simulink model "newBLDCmodel_r2018a"  (R2018a)
settings: Solver=ode4  StartTime=0.0  StopTime=200  FixedStep=.01  MaxStep=.001  RelTol=1e-3
libraries: simulink x8
settings Model: Creator=tdarrah  LastModifiedBy=tdarrah
settings SolverCC: InitialStep=.001  ShapePreserveControl=EnableAll
settings CodeAppCC: StateflowObjectComments=on

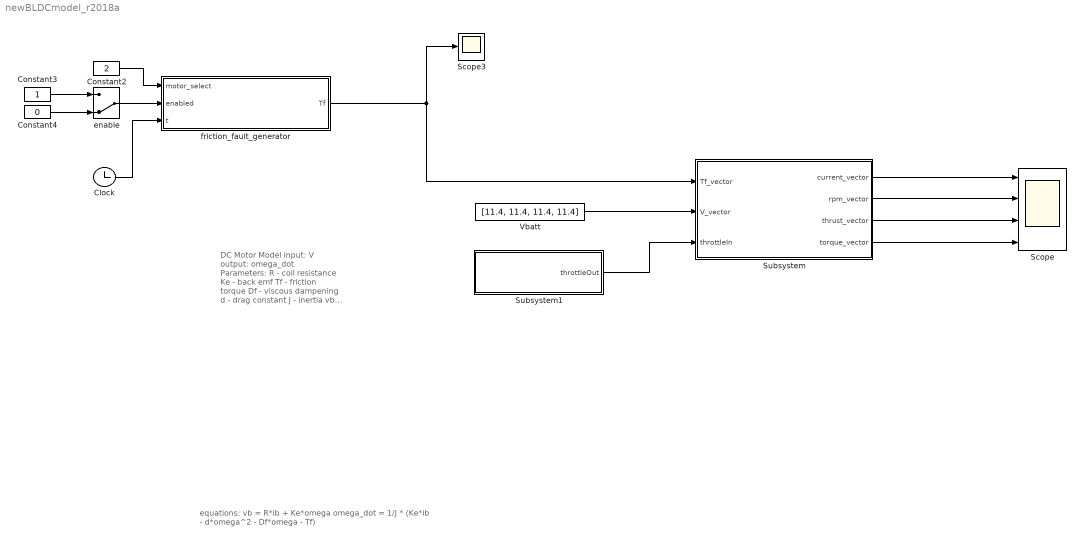
== system newBLDCmodel_r2018a ==
  note: equations:
      |
      | vb = R*ib + Ke*omega
      | omega_dot = 1/J * (Ke*ib - d*omega^2 - Df*omega - Tf)
  note: DC Motor Model
      |
      | input:
      | V
      |
      | output:
      | omega_dot
      |
      | Parameters:
      | R   - coil resistance
      | Ke - back emf
      | Tf  - friction torque
      | Df  - viscous dampening
      | d   - drag constant
      | J   - inertia
      | vb - average battery voltage
      | ib  - average battery current
  Clock : Clock
  Constant2 : Constant  Value=2
  Constant3 : Constant
  Constant4 : Constant  Value=0
  Scope : Scope  NumInputPorts=4
  Scope3 : Scope
  Subsystem : Subsystem
  Subsystem1 : Subsystem
  Vbatt : Constant  Value=[11.4, 11.4, 11.4, 11.4]
  enable : ManualSwitch  CurrentSetting=0
  friction_fault_generator : MATLAB Function  TreatAsAtomicUnit=on
  wires:
  Constant3/1 -> enable/1
  Constant4/1 -> enable/2
  Constant2/1 -> friction_fault_generator/1(motor_select)
  enable/1 -> friction_fault_generator/2(enabled)
  Clock/1 -> friction_fault_generator/3(t)
  friction_fault_generator/1(Tf) -> Subsystem/1(Tf_vector), Scope3/1
  Vbatt/1 -> Subsystem/2(V_vector)
  Subsystem/1(current_vector) -> Scope/1
  Subsystem/2(rpm_vector) -> Scope/2
  Subsystem/3(thrust_vector) -> Scope/3
  Subsystem/4(torque_vector) -> Scope/4
  Subsystem1/1(throttleOut) -> Subsystem/3(throttleIn)

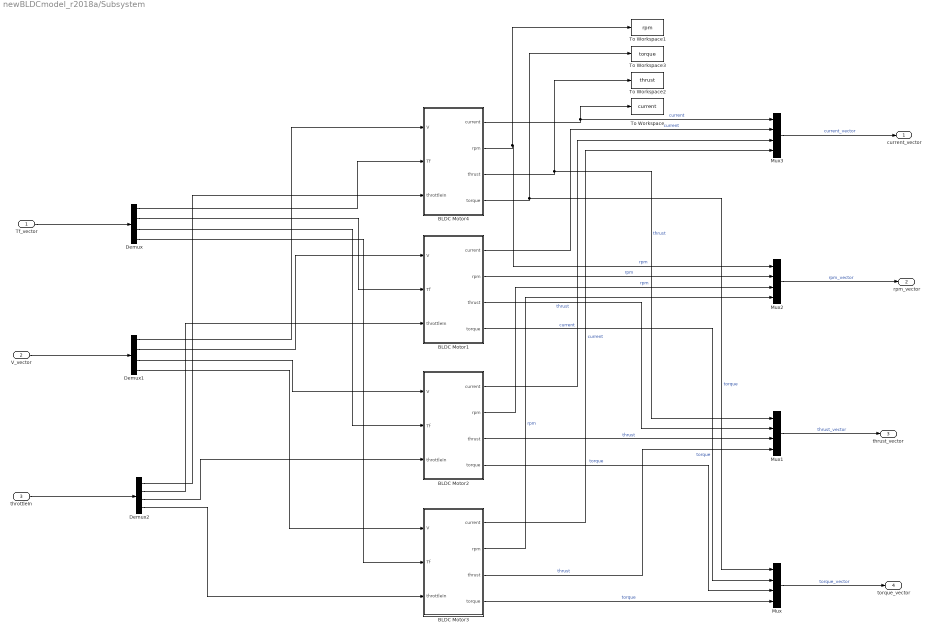
== system newBLDCmodel_r2018a/Subsystem ==
  Tf_vector : Inport
  V_vector : Inport  Port=2
  throttleIn : Inport  Port=3
  BLDC Motor1 : Subsystem
  BLDC Motor2 : Subsystem
  BLDC Motor3 : Subsystem
  BLDC Motor4 : Subsystem
  Demux : Demux
  Demux1 : Demux
  Demux2 : Demux
  Mux{,1..3} (4 alike) : Mux
  To Workspace : ToWorkspace  VariableName=current  SaveFormat=Timeseries  SampleTime=-1
  To Workspace1 : ToWorkspace  VariableName=rpm  SaveFormat=Timeseries  SampleTime=-1
  To Workspace2 : ToWorkspace  VariableName=thrust  SaveFormat=Timeseries  SampleTime=-1
  To Workspace3 : ToWorkspace  VariableName=torque  SaveFormat=Timeseries  SampleTime=-1
  current_vector : Outport
  rpm_vector : Outport  Port=2
  thrust_vector : Outport  Port=3
  torque_vector : Outport  Port=4
  wires:
  BLDC Motor4/2(rpm) -> To Workspace1/1, Mux2/1  "rpm"
  Demux1/3 -> BLDC Motor2/1(V)
  BLDC Motor4/1(current) -> To Workspace/1, Mux3/1  "current"
  BLDC Motor3/3(thrust) -> Mux1/4  "thrust"
  V_vector/1 -> Demux1/1
  Demux1/2 -> BLDC Motor1/1(V)
  BLDC Motor4/3(thrust) -> To Workspace2/1, Mux1/1  "thrust"
  Demux1/4 -> BLDC Motor3/1(V)
  BLDC Motor4/4(torque) -> To Workspace3/1, Mux/1  "torque"
  Mux2/1 -> rpm_vector/1  "rpm_vector"
  Demux/2 -> BLDC Motor1/2(Tf)
  BLDC Motor2/3(thrust) -> Mux1/3  "thrust"
  BLDC Motor1/1(current) -> Mux3/2  "current"
  Tf_vector/1 -> Demux/1
  Demux/1 -> BLDC Motor4/2(Tf)
  BLDC Motor2/1(current) -> Mux3/3  "current"
  Mux3/1 -> current_vector/1  "current_vector"
  BLDC Motor1/3(thrust) -> Mux1/2  "thrust"
  Mux1/1 -> thrust_vector/1  "thrust_vector"
  BLDC Motor2/2(rpm) -> Mux2/3  "rpm"
  Demux/4 -> BLDC Motor3/2(Tf)
  BLDC Motor2/4(torque) -> Mux/3  "torque"
  BLDC Motor1/2(rpm) -> Mux2/2  "rpm"
  Mux/1 -> torque_vector/1  "torque_vector"
  Demux/3 -> BLDC Motor2/2(Tf)
  BLDC Motor1/4(torque) -> Mux/2  "torque"
  BLDC Motor3/1(current) -> Mux3/4  "current"
  Demux1/1 -> BLDC Motor4/1(V)
  BLDC Motor3/4(torque) -> Mux/4  "torque"
  BLDC Motor3/2(rpm) -> Mux2/4  "rpm"
  throttleIn/1 -> Demux2/1
  Demux2/1 -> BLDC Motor4/3(throttleIn)
  Demux2/2 -> BLDC Motor1/3(throttleIn)
  Demux2/3 -> BLDC Motor2/3(throttleIn)
  Demux2/4 -> BLDC Motor3/3(throttleIn)

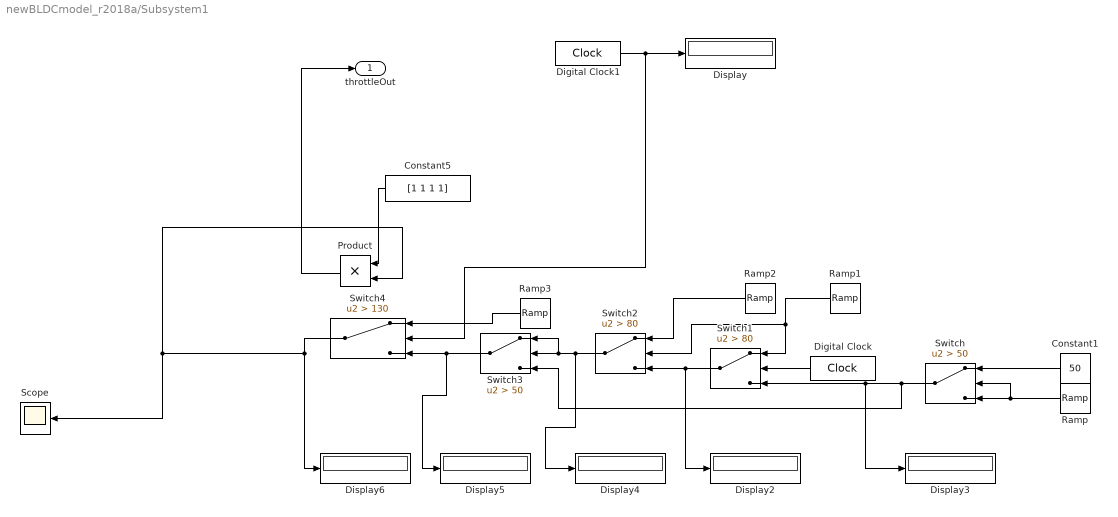
== system newBLDCmodel_r2018a/Subsystem1 ==
  Constant1 : Constant  Value=50
  Constant5 : Constant  Value=[1 1 1 1]
  Digital Clock : DigitalClock
  Digital Clock1 : DigitalClock
  Display{,2..6} (6 alike) : Display
  Product : Product
  Ramp : simulink/Sources/Ramp  slope=1  start=0  InitialOutput=0
  Ramp1 : simulink/Sources/Ramp  slope=2  start=80  InitialOutput=50
  Ramp2 : simulink/Sources/Ramp  slope=-2  start=100  InitialOutput=80
  Ramp3 : simulink/Sources/Ramp  slope=-.63  start=130  InitialOutput=50
  Scope : Scope
  Switch : Switch  Criteria=u2 > Threshold  Threshold=50
  Switch1 : Switch  Criteria=u2 > Threshold  Threshold=80
  Switch2 : Switch  Criteria=u2 > Threshold  Threshold=80
  Switch3 : Switch  Criteria=u2 > Threshold  Threshold=50
  Switch4 : Switch  Criteria=u2 > Threshold  Threshold=130
  throttleOut : Outport
  wires:
  Constant1/1 -> Switch/1
  Product/1 -> throttleOut/1
  Ramp/1 -> Switch/2, Switch/3
  Constant5/1 -> Product/1
  Switch/1 -> Switch3/3, Display3/1, Switch1/3
  Digital Clock/1 -> Switch1/2
  Ramp1/1 -> Switch2/2, Switch1/1
  Switch1/1 -> Display2/1, Switch2/3
  Ramp2/1 -> Switch2/1
  Digital Clock1/1 -> Switch4/2, Display/1
  Switch2/1 -> Display4/1, Switch3/1, Switch3/2
  Switch3/1 -> Display5/1, Switch4/3
  Ramp3/1 -> Switch4/1
  Switch4/1 -> Scope/1, Product/2, Display6/1

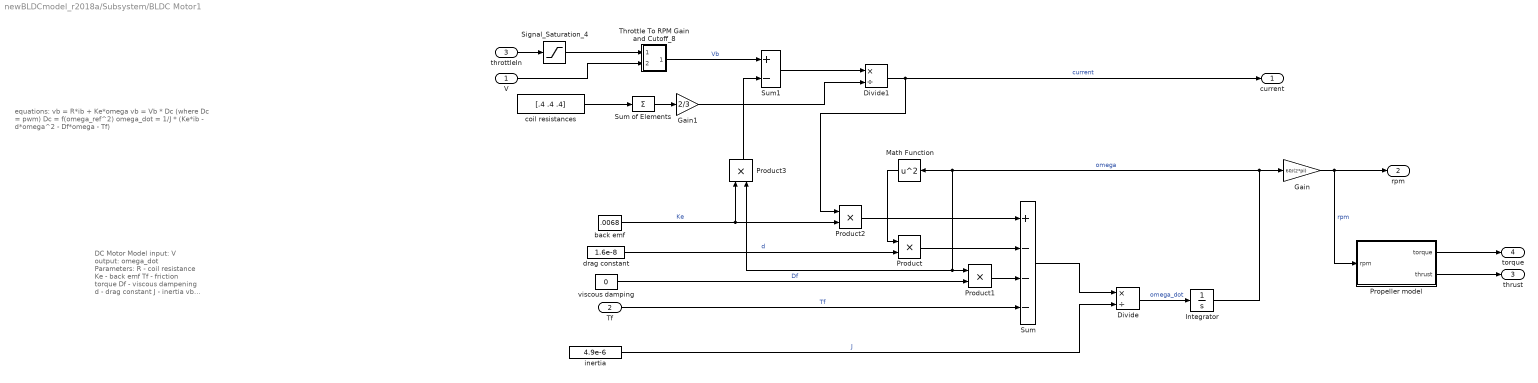
== system newBLDCmodel_r2018a/Subsystem/BLDC Motor1 ==
  note: DC Motor Model
      |
      | input:
      | V
      |
      | output:
      | omega_dot
      |
      | Parameters:
      | R   - coil resistance
      | Ke - back emf
      | Tf  - friction torque
      | Df  - viscous dampening
      | d   - drag constant
      | J   - inertia
      |
      |
      | vb - average battery voltage
      | ib  - average battery current
  note: equations:
      |
      | vb = R*ib + Ke*omega
      | vb = Vb * Dc  (where Dc = pwm)
      | Dc = f(omega_ref^2)
      |
      | omega_dot = 1/J * (Ke*ib - d*omega^2 - Df*omega - Tf)
  V : Inport
  Tf : Inport  Port=2
  throttleIn : Inport  Port=3
  Divide : Product  Inputs=*/
  Divide1 : Product  Inputs=*/
  Gain : Gain  Gain=60/(2*pi)
  Gain1 : Gain  Gain=2/3
  Integrator : Integrator
  Math Function : Math  Operator=square  SaturateOnIntegerOverflow=on
  Product{,1..3} (4 alike) : Product
  "Propeller model " : MATLAB Function  TreatAsAtomicUnit=on
  Signal_Saturation_4 : Saturate  UpperLimit=100  LowerLimit=0
  Sum : Sum  Inputs=+---
  Sum of Elements : Sum  Inputs=+
  Sum1 : Sum  Inputs=+-
  Throttle To RPM Gain and Cutoff_8 : Subsystem
  back emf : Constant  Value=.0068
  coil resistances : Constant  Value=[.4 .4 .4]
  drag constant : Constant  Value=1.6e-8
  inertia : Constant  Value=4.9e-6
  viscous damping : Constant  Value=0
  current : Outport
  rpm : Outport  Port=2
  thrust : Outport  Port=3
  torque : Outport  Port=4
  wires:
  Divide/1 -> Integrator/1  "omega_dot"
  Integrator/1 -> Math Function/1, Product1/1, Product3/2, Gain/1  "omega"
  Gain/1 -> rpm/1, "Propeller model "/1(rpm)  "rpm"
  inertia/1 -> Divide/2  "J"
  drag constant/1 -> Product/2  "d"
  Math Function/1 -> Product/1
  viscous damping/1 -> Product1/2  "Df"
  Tf/1 -> Sum/4  "Tf"
  back emf/1 -> Product3/1, Product2/2  "Ke"
  Product2/1 -> Sum/1
  Divide1/1 -> Product2/1, current/1  "current"
  V/1 -> Throttle To RPM Gain and Cutoff_8/2(Vs)
  Product3/1 -> Sum1/2
  Sum1/1 -> Divide1/1
  Gain1/1 -> Divide1/2
  "Propeller model "/2(thrust) -> thrust/1
  "Propeller model "/1(torque) -> torque/1
  Product1/1 -> Sum/3
  Product/1 -> Sum/2
  Sum/1 -> Divide/1
  coil resistances/1 -> Sum of Elements/1
  Sum of Elements/1 -> Gain1/1
  throttleIn/1 -> Signal_Saturation_4/1
  Signal_Saturation_4/1 -> Throttle To RPM Gain and Cutoff_8/1(In5)
  Throttle To RPM Gain and Cutoff_8/1(Out5) -> Sum1/1  "Vb"

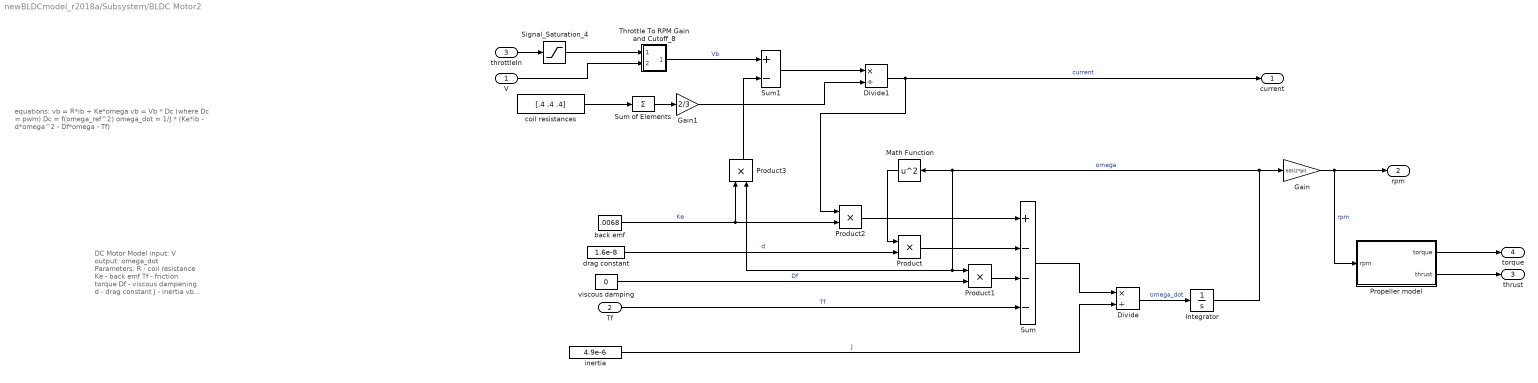
== system newBLDCmodel_r2018a/Subsystem/BLDC Motor2 ==
  note: DC Motor Model
      |
      | input:
      | V
      |
      | output:
      | omega_dot
      |
      | Parameters:
      | R   - coil resistance
      | Ke - back emf
      | Tf  - friction torque
      | Df  - viscous dampening
      | d   - drag constant
      | J   - inertia
      |
      |
      | vb - average battery voltage
      | ib  - average battery current
  note: equations:
      |
      | vb = R*ib + Ke*omega
      | vb = Vb * Dc  (where Dc = pwm)
      | Dc = f(omega_ref^2)
      |
      | omega_dot = 1/J * (Ke*ib - d*omega^2 - Df*omega - Tf)
  V : Inport
  Tf : Inport  Port=2
  throttleIn : Inport  Port=3
  Divide : Product  Inputs=*/
  Divide1 : Product  Inputs=*/
  Gain : Gain  Gain=60/(2*pi)
  Gain1 : Gain  Gain=2/3
  Integrator : Integrator
  Math Function : Math  Operator=square  SaturateOnIntegerOverflow=on
  Product{,1..3} (4 alike) : Product
  "Propeller model " : MATLAB Function  TreatAsAtomicUnit=on
  Signal_Saturation_4 : Saturate  UpperLimit=100  LowerLimit=0
  Sum : Sum  Inputs=+---
  Sum of Elements : Sum  Inputs=+
  Sum1 : Sum  Inputs=+-
  Throttle To RPM Gain and Cutoff_8 : Subsystem
  back emf : Constant  Value=.0068
  coil resistances : Constant  Value=[.4 .4 .4]
  drag constant : Constant  Value=1.6e-8
  inertia : Constant  Value=4.9e-6
  viscous damping : Constant  Value=0
  current : Outport
  rpm : Outport  Port=2
  thrust : Outport  Port=3
  torque : Outport  Port=4
  wires:
  Divide/1 -> Integrator/1  "omega_dot"
  Integrator/1 -> Math Function/1, Product1/1, Product3/2, Gain/1  "omega"
  Gain/1 -> rpm/1, "Propeller model "/1(rpm)  "rpm"
  inertia/1 -> Divide/2  "J"
  drag constant/1 -> Product/2  "d"
  Math Function/1 -> Product/1
  viscous damping/1 -> Product1/2  "Df"
  Tf/1 -> Sum/4  "Tf"
  back emf/1 -> Product3/1, Product2/2  "Ke"
  Product2/1 -> Sum/1
  Divide1/1 -> Product2/1, current/1  "current"
  V/1 -> Throttle To RPM Gain and Cutoff_8/2(Vs)
  Product3/1 -> Sum1/2
  Sum1/1 -> Divide1/1
  Gain1/1 -> Divide1/2
  "Propeller model "/2(thrust) -> thrust/1
  "Propeller model "/1(torque) -> torque/1
  Product1/1 -> Sum/3
  Product/1 -> Sum/2
  Sum/1 -> Divide/1
  coil resistances/1 -> Sum of Elements/1
  Sum of Elements/1 -> Gain1/1
  throttleIn/1 -> Signal_Saturation_4/1
  Signal_Saturation_4/1 -> Throttle To RPM Gain and Cutoff_8/1(In5)
  Throttle To RPM Gain and Cutoff_8/1(Out5) -> Sum1/1  "Vb"

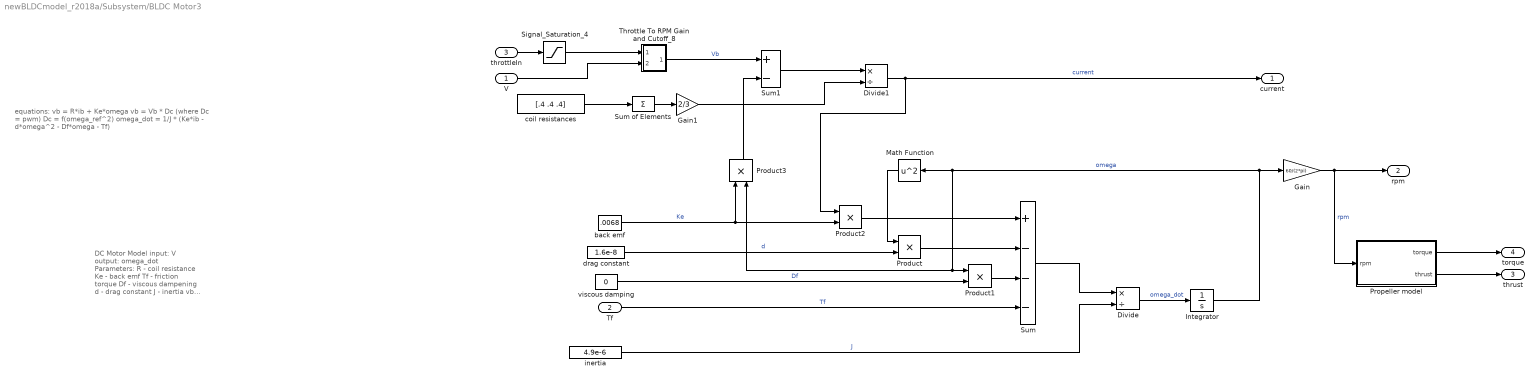
== system newBLDCmodel_r2018a/Subsystem/BLDC Motor3 ==
  note: DC Motor Model
      |
      | input:
      | V
      |
      | output:
      | omega_dot
      |
      | Parameters:
      | R   - coil resistance
      | Ke - back emf
      | Tf  - friction torque
      | Df  - viscous dampening
      | d   - drag constant
      | J   - inertia
      |
      |
      | vb - average battery voltage
      | ib  - average battery current
  note: equations:
      |
      | vb = R*ib + Ke*omega
      | vb = Vb * Dc  (where Dc = pwm)
      | Dc = f(omega_ref^2)
      |
      | omega_dot = 1/J * (Ke*ib - d*omega^2 - Df*omega - Tf)
  V : Inport
  Tf : Inport  Port=2
  throttleIn : Inport  Port=3
  Divide : Product  Inputs=*/
  Divide1 : Product  Inputs=*/
  Gain : Gain  Gain=60/(2*pi)
  Gain1 : Gain  Gain=2/3
  Integrator : Integrator
  Math Function : Math  Operator=square  SaturateOnIntegerOverflow=on
  Product{,1..3} (4 alike) : Product
  "Propeller model " : MATLAB Function  TreatAsAtomicUnit=on
  Signal_Saturation_4 : Saturate  UpperLimit=100  LowerLimit=0
  Sum : Sum  Inputs=+---
  Sum of Elements : Sum  Inputs=+
  Sum1 : Sum  Inputs=+-
  Throttle To RPM Gain and Cutoff_8 : Subsystem
  back emf : Constant  Value=.0068
  coil resistances : Constant  Value=[.4 .4 .4]
  drag constant : Constant  Value=1.6e-8
  inertia : Constant  Value=4.9e-6
  viscous damping : Constant  Value=0
  current : Outport
  rpm : Outport  Port=2
  thrust : Outport  Port=3
  torque : Outport  Port=4
  wires:
  Divide/1 -> Integrator/1  "omega_dot"
  Integrator/1 -> Math Function/1, Product1/1, Product3/2, Gain/1  "omega"
  Gain/1 -> rpm/1, "Propeller model "/1(rpm)  "rpm"
  inertia/1 -> Divide/2  "J"
  drag constant/1 -> Product/2  "d"
  Math Function/1 -> Product/1
  viscous damping/1 -> Product1/2  "Df"
  Tf/1 -> Sum/4  "Tf"
  back emf/1 -> Product3/1, Product2/2  "Ke"
  Product2/1 -> Sum/1
  Divide1/1 -> Product2/1, current/1  "current"
  V/1 -> Throttle To RPM Gain and Cutoff_8/2(Vs)
  Product3/1 -> Sum1/2
  Sum1/1 -> Divide1/1
  Gain1/1 -> Divide1/2
  "Propeller model "/2(thrust) -> thrust/1
  "Propeller model "/1(torque) -> torque/1
  Product1/1 -> Sum/3
  Product/1 -> Sum/2
  Sum/1 -> Divide/1
  coil resistances/1 -> Sum of Elements/1
  Sum of Elements/1 -> Gain1/1
  throttleIn/1 -> Signal_Saturation_4/1
  Signal_Saturation_4/1 -> Throttle To RPM Gain and Cutoff_8/1(In5)
  Throttle To RPM Gain and Cutoff_8/1(Out5) -> Sum1/1  "Vb"

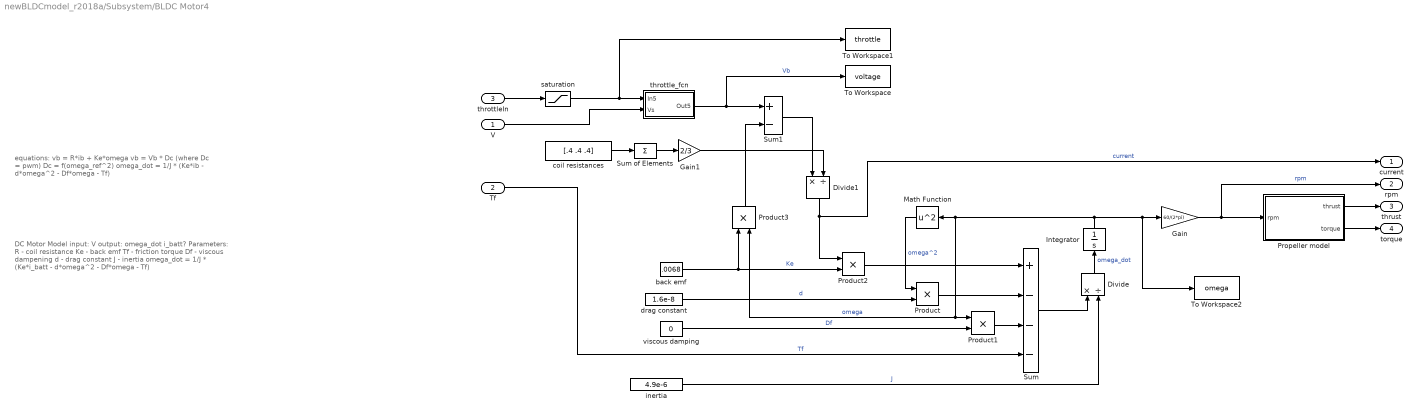
== system newBLDCmodel_r2018a/Subsystem/BLDC Motor4 ==
  note: DC Motor Model
      |
      | input:
      | V
      |
      | output:
      | omega_dot
      | i_batt?
      |
      |
      | Parameters:
      | R   - coil resistance
      | Ke - back emf
      | Tf  - friction torque
      | Df  - viscous dampening
      | d   - drag constant
      | J   - inertia
      |
      | omega_dot = 1/J * (Ke*i_batt - d*omega^2 - Df*omega - Tf)
  note: equations:
      |
      | vb = R*ib + Ke*omega
      | vb = Vb * Dc  (where Dc = pwm)
      | Dc = f(omega_ref^2)
      |
      | omega_dot = 1/J * (Ke*ib - d*omega^2 - Df*omega - Tf)
  V : Inport
  Tf : Inport  Port=2
  throttleIn : Inport  Port=3
  Divide : Product  Inputs=*/
  Divide1 : Product  Inputs=*/
  Gain : Gain  Gain=60/(2*pi)
  Gain1 : Gain  Gain=2/3
  Integrator : Integrator
  Math Function : Math  Operator=square  SaturateOnIntegerOverflow=on
  Product{,1..3} (4 alike) : Product
  "Propeller model " : MATLAB Function  TreatAsAtomicUnit=on
  Sum : Sum  Inputs=+---
  Sum of Elements : Sum  Inputs=+
  Sum1 : Sum  Inputs=+-
  To Workspace : ToWorkspace  VariableName=voltage  SaveFormat=Timeseries  SampleTime=-1
  To Workspace1 : ToWorkspace  VariableName=throttle  SaveFormat=Timeseries  SampleTime=-1
  To Workspace2 : ToWorkspace  VariableName=omega  SaveFormat=Timeseries  SampleTime=-1
  back emf : Constant  Value=.0068
  coil resistances : Constant  Value=[.4 .4 .4]
  drag constant : Constant  Value=1.6e-8
  inertia : Constant  Value=4.9e-6
  saturation : Saturate  UpperLimit=100  LowerLimit=0
  throttle_fcn : Subsystem
  viscous damping : Constant  Value=0
  current : Outport
  rpm : Outport  Port=2
  thrust : Outport  Port=3
  torque : Outport  Port=4
  wires:
  Divide/1 -> Integrator/1  "omega_dot"
  Integrator/1 -> To Workspace2/1, Gain/1, Math Function/1, Product1/1, Product3/2  "omega"
  Gain/1 -> "Propeller model "/1(rpm), rpm/1  "rpm"
  inertia/1 -> Divide/2  "J"
  drag constant/1 -> Product/2  "d"
  Math Function/1 -> Product/1  "omega^2"
  viscous damping/1 -> Product1/2  "Df"
  Tf/1 -> Sum/4  "Tf"
  back emf/1 -> Product3/1, Product2/2  "Ke"
  Product2/1 -> Sum/1
  Divide1/1 -> current/1, Product2/1  "current"
  V/1 -> throttle_fcn/2(Vs)
  Product3/1 -> Sum1/2
  Sum1/1 -> Divide1/1
  Gain1/1 -> Divide1/2
  "Propeller model "/1(thrust) -> thrust/1
  "Propeller model "/2(torque) -> torque/1
  Product1/1 -> Sum/3
  Product/1 -> Sum/2
  Sum/1 -> Divide/1
  coil resistances/1 -> Sum of Elements/1
  Sum of Elements/1 -> Gain1/1
  throttleIn/1 -> saturation/1
  throttle_fcn/1(Out5) -> To Workspace/1, Sum1/1  "Vb"
  saturation/1 -> To Workspace1/1, throttle_fcn/1(In5)

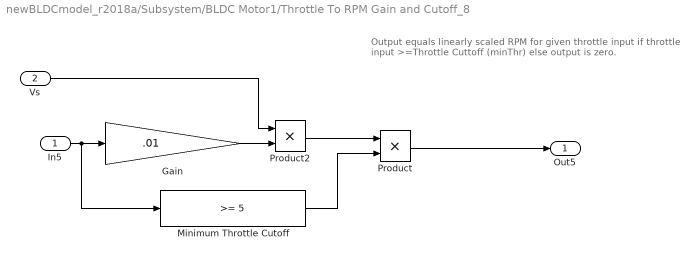
== system newBLDCmodel_r2018a/Subsystem/BLDC Motor1/Throttle To RPM Gain and Cutoff_8 ==
  note: Output equals linearly scaled RPM
      | for given throttle input if throttle input >=Throttle Cuttoff (minThr)
      | else output is zero.
  In5 : Inport
  Vs : Inport  Port=2
  Gain : Gain  Gain=.01
  Minimum Throttle Cutoff : simulink/Logic and Bit Operations/Compare To Constant  relop=>=  const=5  OutDataTypeStr=uint8
  Product : Product
  Product2 : Product
  Out5 : Outport
  wires:
  Minimum Throttle Cutoff/1 -> Product/2
  Product/1 -> Out5/1
  In5/1 -> Gain/1, Minimum Throttle Cutoff/1
  Gain/1 -> Product2/2
  Product2/1 -> Product/1
  Vs/1 -> Product2/1

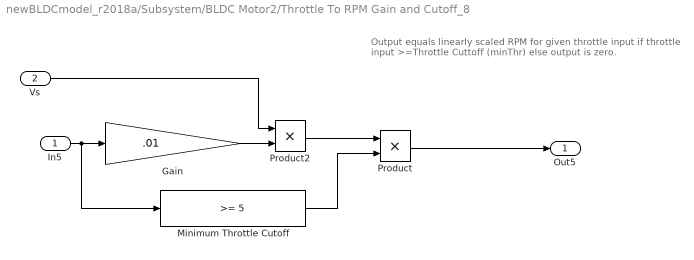
== system newBLDCmodel_r2018a/Subsystem/BLDC Motor2/Throttle To RPM Gain and Cutoff_8 ==
  note: Output equals linearly scaled RPM
      | for given throttle input if throttle input >=Throttle Cuttoff (minThr)
      | else output is zero.
  In5 : Inport
  Vs : Inport  Port=2
  Gain : Gain  Gain=.01
  Minimum Throttle Cutoff : simulink/Logic and Bit Operations/Compare To Constant  relop=>=  const=5  OutDataTypeStr=uint8
  Product : Product
  Product2 : Product
  Out5 : Outport
  wires:
  Minimum Throttle Cutoff/1 -> Product/2
  Product/1 -> Out5/1
  In5/1 -> Gain/1, Minimum Throttle Cutoff/1
  Gain/1 -> Product2/2
  Product2/1 -> Product/1
  Vs/1 -> Product2/1

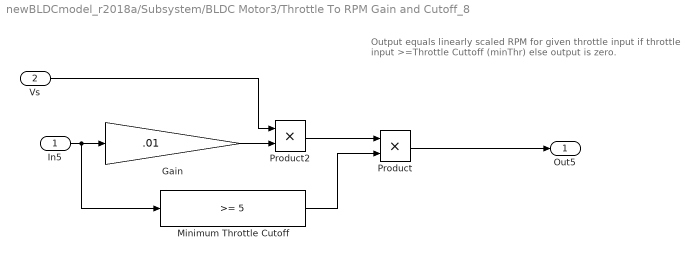
== system newBLDCmodel_r2018a/Subsystem/BLDC Motor3/Throttle To RPM Gain and Cutoff_8 ==
  note: Output equals linearly scaled RPM
      | for given throttle input if throttle input >=Throttle Cuttoff (minThr)
      | else output is zero.
  In5 : Inport
  Vs : Inport  Port=2
  Gain : Gain  Gain=.01
  Minimum Throttle Cutoff : simulink/Logic and Bit Operations/Compare To Constant  relop=>=  const=5  OutDataTypeStr=uint8
  Product : Product
  Product2 : Product
  Out5 : Outport
  wires:
  Minimum Throttle Cutoff/1 -> Product/2
  Product/1 -> Out5/1
  In5/1 -> Gain/1, Minimum Throttle Cutoff/1
  Gain/1 -> Product2/2
  Product2/1 -> Product/1
  Vs/1 -> Product2/1

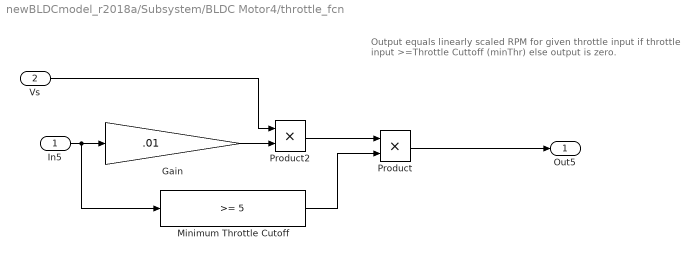
== system newBLDCmodel_r2018a/Subsystem/BLDC Motor4/throttle_fcn ==
  note: Output equals linearly scaled RPM
      | for given throttle input if throttle input >=Throttle Cuttoff (minThr)
      | else output is zero.
  In5 : Inport
  Vs : Inport  Port=2
  Gain : Gain  Gain=.01
  Minimum Throttle Cutoff : simulink/Logic and Bit Operations/Compare To Constant  relop=>=  const=5  OutDataTypeStr=uint8
  Product : Product
  Product2 : Product
  Out5 : Outport
  wires:
  Minimum Throttle Cutoff/1 -> Product/2
  Product/1 -> Out5/1
  In5/1 -> Gain/1, Minimum Throttle Cutoff/1
  Gain/1 -> Product2/2
  Product2/1 -> Product/1
  Vs/1 -> Product2/1

== matlab function newBLDCmodel_r2018a/Subsystem/BLDC Motor1/Propeller model  ==
  data: torque output; rpm input; thrust output
function [torque,thrust] = fcn(rpm)
% angular_velocity in rpm

%coefficient of thrust, empirically derived
coef_t = 2*(10^-15)*rpm^3 - 4*(10^-11)*rpm^2 + 3*(10^-7)*rpm + .1013;
%thrust = coef_t * density of air * velocity^2 * propeller diameter (m) ^4
thrust = coef_t*1.225*(rpm/60)^2*.2^4;
% empirically derived
torque = 4*(10^-14)*rpm^3 +  8*(10^-12)*rpm^2 + 3*(10^-6)*rpm;
end

== matlab function newBLDCmodel_r2018a/Subsystem/BLDC Motor2/Propeller model  ==
  data: torque output; rpm input; thrust output
function [torque,thrust] = fcn(rpm)
% angular_velocity in rpm

%coefficient of thrust, empirically derived
coef_t = 2*(10^-15)*rpm^3 - 4*(10^-11)*rpm^2 + 3*(10^-7)*rpm + .1013;
%thrust = coef_t * density of air * velocity^2 * propeller diameter (m) ^4
thrust = coef_t*1.225*(rpm/60)^2*.2^4;
% empirically derived
torque = 4*(10^-14)*rpm^3 +  8*(10^-12)*rpm^2 + 3*(10^-6)*rpm;
end

== matlab function newBLDCmodel_r2018a/Subsystem/BLDC Motor4/Propeller model  ==
  data: thrust output; torque output; rpm input
function [thrust,torque] = fcn(rpm)
% angular_velocity in rpm

%coefficient of thrust, empirically derived
coef_t = 2*(10^-15)*rpm^3 - 4*(10^-11)*rpm^2 + 3*(10^-7)*rpm + .1013;
%thrust = coef_t * density of air * velocity^2 * propeller diameter (m) ^4
thrust = coef_t*1.225*(rpm/60)^2*.2^4;
% empirically derived
torque = 4*(10^-14)*rpm^3 +  8*(10^-12)*rpm^2 + 3*(10^-6)*rpm;
end

== matlab function newBLDCmodel_r2018a/Subsystem/BLDC Motor3/Propeller model  ==
  data: torque output; rpm input; thrust output
function [torque,thrust] = fcn(rpm)
% angular_velocity in rpm

%coefficient of thrust, empirically derived
coef_t = 2*(10^-15)*rpm^3 - 4*(10^-11)*rpm^2 + 3*(10^-7)*rpm + .1013;
%thrust = coef_t * density of air * velocity^2 * propeller diameter (m) ^4
thrust = coef_t*1.225*(rpm/60)^2*.2^4;
% empirically derived
torque = 4*(10^-14)*rpm^3 +  8*(10^-12)*rpm^2 + 3*(10^-6)*rpm;
end

== matlab function newBLDCmodel_r2018a/friction_fault_generator ==
  settings: updateMethod=DISCRETE
  data: motor_select input; enabled input; t input; Tf output
function Tf = friction_fault_generator(motor_select, enabled, t)

Tf = [1e-8,1e-8,1e-8,1e-8];

if enabled == 1
    Tf(motor_select) = Tf(motor_select) + abs(normrnd(0, 1e-5 * t));
end
